simulink model "Model_TranslationEngine64"  (R2022b)
settings: Solver=FixedStepDiscrete  StartTime=0.0  StopTime=5  RelTol=1e-3  EnableMultiTasking=on
InitFcn:
  | % Initialize model
  | ModelSettings=BTConfig.GetModelSettings();
  | 
  | ModelSettings.Validate();
  | 
  | ModelInit;
  | 
  | 
  | % load library data
  | GainLibrary_data;
  | % Load saved values from partition process
  | CapturedConstMask.LoadMapFromFile(bdroot)
StartFcn:
  | % make sure all the simulated RTC requests are found
  | %RTC_SIM_OBJ.ValidateREQs();
undefined symbols (not defined in the file or in its folder): AA, BPLP, Column, NumHFRefBPF, NumHFRefLPF, NumMusicChannels, Row, VolumeMuteConfig
libraries: TuneVar x925, TOP x490, FeaturePath x111, CapturedConstLib x52
(part 5 of 34)

== system Model_TranslationEngine64/ModelPreAmp/DecRate/AudioPilot35/EntertainmentLevelDetection/PreProcessing ==
  FeaturePath : FeaturePath/FeaturePath  FeatureName=LevelDetect  IsGroup=off  GroupNumber=-1  IsModule=off  TriggerInit=[565 224 680 331]
      settings: SourceProductName=Bose Talaria
  MusicDelay : Subsystem
  PreEmphasisShelfFilter : Subsystem  LoadFcn="fprintf(\"\\n ''%s'' block does not support BTC and hence, it will be deprecated soon. Please replace all the active instances of \"\"PooliirwithNonTrivialTranslations\"\" with an equivalent BTC block.\", gcb);"  mask(Bose Pool IIR){maxNumStages=NumInputChannels * Config.ShelfNumStages, numStages=repmat(Config.ShelfNumStages,NumInputChannels,1), sosCoefficients=repmat(Config.ShelfSos,NumInputChannels,1), alias='Default', variantType=Config.LevDetPreEmpPooliirVariant, FeatureName=Preemphasis}
      mask prompts: maxNumStages "Maximum number of stages"; numStages "Number of stages per channel"; sosCoefficients "Coefficient pool"; variantType "Variant"; FeatureName "Filter name/purpose"
      mask init:
      | blkh = gcbh;
      | % Copy discrete mask parameters into a classdef object
      | InnerLinkConfig = PoolIirTunableConfig;
      | InnerLinkConfig.MaxNumStages = maxNumStages;
      | InnerLinkConfig.DefaultNumStages = numStages;
      | InnerLinkConfig.DefaultSosCoefficients = sosCoefficients;
      | InnerLinkConfig.Alias = alias;
      | if(isa(variantType, 'char'))
      |     InnerLinkConfig.SelectVariant(variantType);
      | else
      |     error("Please specify the variant in a character format for ''%s''", gcb);
      | end
      mask TypeOptions FeatureName: InnerLink/FeatureName
      mask Display:
      | [path,w,h] = IconIIR_Mask();
      | 
      | % work in pixels since the icon does not scale
      | pos = get(gcbh,'position');
      | bw = pos(3) - pos(1);
      | bh = pos(4) - pos(2);
      | 
      | % Draw centered icon
      | xAdj = bw/2 - w/2;
      | yAdj = bh/2 - h/2 + 4;
      | for i=1:length(path)
      | %     patch(path(i).x+xAdj, path(i).y+yAdj, path(i).rgb);
      |     plot(path(i).x+xAdj, path(i).y+yAdj);
      | end
      | 
      | % Anchor the corners of the coordinate system
      | patch(0,0,[1 1 1]);
      | patch(bw,bh,[1 1 1]);
      | 
      | % Display some text
      | text(bw/2, 1,'Pool IIR', ...
      |     'horizontalAlignment','center', ...
      |     'VerticalAlignment','bottom');
  SysMax : Subsystem  mask(Talaria Trivial Tune TOP){TriggerInit=[215 414 420 476], TopName=SysMaxDbspl, TuneName=SysMaxDbspl, DataTypeOut=single, MaskValue=Config.MaxDbspl, TunabilityNumber=1, MinValue=[], MaxValue=[], BankNumber=0, PreOverlay=false, PostOverlay=false, UseSameName=on}
      mask prompts: TriggerInit "Hidden: MoveFcn redraw"; TopName "Name:"; TuneName "Name of TuneVar:"; DataTypeOut "Data type:"; MaskValue "Default Value:"; TunabilityNumber "Tunability:"; MinValue "Min Value:"; MaxValue "Max Value:"; BankNumber "Target memory bank number:"; PreOverlay "Requires pre-overlay action:"; PostOverlay "Requires post-overlay action:"; UseSameName "Use same name for tune variable and TOP"
      mask help: The TuneTOP block encapsultes a Target Overlay Parameter, a Tune Variable, and a Trivial Translation between them.
      mask init:
      | [ok,activeTopPath,activeTunePath] = TuneTOP_Mask.Init(gcbh);
      settings: MoveFcn=TuneTOP_Mask.CB_TriggerInit(gcbh);
      mask Callback TriggerInit: TuneTOP_Mask.CB_TriggerInit(gcbh);
      mask TypeOptions TopName: TOP/TopName
      mask TypeOptions TuneName: Tune Variable/TuneName
      mask TypeOptions DataTypeOut: TOP/DataTypeOut
      mask TypeOptions MaskValue: Tune Variable/MaskValue
      mask TypeOptions TunabilityNumber: Tune Variable/TunabilityNumber
      mask Callback TunabilityNumber: TuneVarMask.CB_TunabilityNumber(gcbh);
      mask TypeOptions MinValue: Tune Variable/MinValue
      mask TypeOptions MaxValue: Tune Variable/MaxValue
      mask TypeOptions BankNumber: TOP/BankNumber
      mask TypeOptions PreOverlay: TOP/PreOverlay
      mask TypeOptions PostOverlay: TOP/PostOverlay
      mask Callback UseSameName: TuneTOP_Mask.CB_UseSameName(gcbh);
      mask DialogControl toolPanel Prompt: Tuning Tool Hints
      mask DialogControl DescriptionGroup Prompt: Description
      mask DialogControl EditDescription Prompt: Edit Description
      mask DialogControl EditDescription Callback: TuneTOP_Mask.CB_EditDescription(gcbh);
      mask DialogControl TunabilityText Prompt: Easy: Changes nearly every tuning.
      mask DialogControl AdvancedPanel Prompt: Advanced
      mask DialogControl ConvertToFullTranslation Prompt: Irreversible conversion to full translation
      mask DialogControl ConvertToFullTranslation Callback: TuneTOP_Mask.CB_ConvertToFullTranslation(gcbh);
      mask DialogControl ErrorContainer Prompt: Error Messages
      mask Display:
      | % retrieve icon definition
      | [path,w,h] = TuneTOP_Mask.Icon();
      | 
      | % retrieve the block's pixel size
      | pos = get(gcbh,'position');
      | bw = pos(3) - pos(1);
      | bh = pos(4) - pos(2);
      | 
      | % draw centered icon
      | xAdj = bw/2 - w/2 + 5;
      | yAdj = bh/2 - h/2 + 4;
      | for i=1:length(path)
      | 	patch(path(i).x+xAdj, path(i).y+yAdj, path(i).rgb);
      | end
      | 
      | % show the top name or an X
      | if (exist('ok','var') && ok)
      | 	text(bw*0.5, bh*0.2, activeTopPath, 'horizontalAlignment', 'center');
      | 	patch(0,0,[1 1 1]);
      | 	patch(bw,bh,[1 1 1]);
      | else
      | 	tx=bw*0.03;
      | 	ty=bh*0.03;
      | 	patch([0 tx bw bw-tx], [ty 0 bh-ty bh], [1 0 0]);
      | 	patch([0 bw-tx bw tx], [bh-ty 0 ty bh], [1 0 0]);
      | end

== system Model_TranslationEngine64/ModelPreAmp/DecRate/AudioPilot35/Volume/Index2DbTable ==
  TOP_GainDB : TOP/TOP  TriggerInit=[635 177 785 233]  TopName=Table_dB  DataTypeOut=Inherit: Same as input  BankNumber=Config.BankNumber  PreOverlay=false  PostOverlay=false  Role=Automatic
      settings: SourceProductName=Bose Talaria
  TOP_Index : TOP/TOP  TriggerInit=[635 97 785 153]  TopName=Table_Idx  DataTypeOut=Inherit: Same as input  BankNumber=Config.BankNumber  PreOverlay=false  PostOverlay=false  Role=Automatic
      settings: SourceProductName=Bose Talaria
  TranslateTrigger1 : TuneVar/TranslateTrigger  TriggerInit=[491 -5 529 45]
      settings: SourceProductName=Bose Talaria
  TuneTOP : Subsystem  Description=Variable limits the maximum *dB offset* which will be applied to the gain as part of table lookup. It does *not* directly impact the maximum gain applied, only the maximum dB offset.  mask(Talaria Trivial Tune TOP){TriggerInit=[670 347 840 403], TopName=maxgain, TuneName=maxgain, DataTypeOut=single, MaskValue=Config.DefaultMaxDbOffset, TunabilityNumber=1, MinValue=[], MaxValue=[], BankNumber=0, PreOverlay=false, PostOverlay=false, UseSameName=on}
      mask prompts: TriggerInit "Hidden: MoveFcn redraw"; TopName "Name:"; TuneName "Name of TuneVar:"; DataTypeOut "Data type:"; MaskValue "Default Value:"; TunabilityNumber "Tunability:"; MinValue "Min Value:"; MaxValue "Max Value:"; BankNumber "Target memory bank number:"; PreOverlay "Requires pre-overlay action:"; PostOverlay "Requires post-overlay action:"; UseSameName "Use same name for tune variable and TOP"
      mask help: The TuneTOP block encapsultes a Target Overlay Parameter, a Tune Variable, and a Trivial Translation between them.
      mask init:
      | [ok,activeTopPath,activeTunePath] = TuneTOP_Mask.Init(gcbh);
      settings: MoveFcn=TuneTOP_Mask.CB_TriggerInit(gcbh);
      mask Callback TriggerInit: TuneTOP_Mask.CB_TriggerInit(gcbh);
      mask TypeOptions TopName: TOP/TopName
      mask TypeOptions TuneName: Tune Variable/TuneName
      mask TypeOptions DataTypeOut: TOP/DataTypeOut
      mask TypeOptions MaskValue: Tune Variable/MaskValue
      mask TypeOptions TunabilityNumber: Tune Variable/TunabilityNumber
      mask Callback TunabilityNumber: TuneVarMask.CB_TunabilityNumber(gcbh);
      mask TypeOptions MinValue: Tune Variable/MinValue
      mask TypeOptions MaxValue: Tune Variable/MaxValue
      mask TypeOptions BankNumber: TOP/BankNumber
      mask TypeOptions PreOverlay: TOP/PreOverlay
      mask TypeOptions PostOverlay: TOP/PostOverlay
      mask Callback UseSameName: TuneTOP_Mask.CB_UseSameName(gcbh);
      mask DialogControl toolPanel Prompt: Tuning Tool Hints
      mask DialogControl DescriptionGroup Prompt: Description
      mask DialogControl EditDescription Prompt: Edit Description
      mask DialogControl EditDescription Callback: TuneTOP_Mask.CB_EditDescription(gcbh);
      mask DialogControl TunabilityText Prompt: Easy: Changes nearly every tuning.
      mask DialogControl AdvancedPanel Prompt: Advanced
      mask DialogControl ConvertToFullTranslation Prompt: Irreversible conversion to full translation
      mask DialogControl ConvertToFullTranslation Callback: TuneTOP_Mask.CB_ConvertToFullTranslation(gcbh);
      mask DialogControl ErrorContainer Prompt: Error Messages
      mask Display:
      | % retrieve icon definition
      | [path,w,h] = TuneTOP_Mask.Icon();
      | 
      | % retrieve the block's pixel size
      | pos = get(gcbh,'position');
      | bw = pos(3) - pos(1);
      | bh = pos(4) - pos(2);
      | 
      | % draw centered icon
      | xAdj = bw/2 - w/2 + 5;
      | yAdj = bh/2 - h/2 + 4;
      | for i=1:length(path)
      | 	patch(path(i).x+xAdj, path(i).y+yAdj, path(i).rgb);
      | end
      | 
      | % show the top name or an X
      | if (exist('ok','var') && ok)
      | 	text(bw*0.5, bh*0.2, activeTopPath, 'horizontalAlignment', 'center');
      | 	patch(0,0,[1 1 1]);
      | 	patch(bw,bh,[1 1 1]);
      | else
      | 	tx=bw*0.03;
      | 	ty=bh*0.03;
      | 	patch([0 tx bw bw-tx], [ty 0 bh-ty bh], [1 0 0]);
      | 	patch([0 bw-tx bw tx], [bh-ty 0 ty bh], [1 0 0]);
      | end
  TuneVar_Table : TuneVar/TuneVar  Description=|  TuneName=Table  SpecifyMaxSize=on  VariableDim=1 (Row)  MaxSize=[Config.MaximumTablePoints 2]  TunabilityNumber=2  MinValue=[0;-100]  MaxValue=[1;0]  TriggerInit=[190 140 360 190]  MaskValue=Config.DefaultTable
      | <HTML>Gain table maps index to gain.
      | The index values are <FONT color="red">normalized</Font> floats between 0 and 1 while the gains are in dB (i.e. 0 implies no attenuation).
      | </html>
      settings: SourceProductName=Bose Talaria
  table translation : MATLAB Function  TreatAsAtomicUnit=on
  wires:
  table translation/2(Table_dB) -> TOP_GainDB/1
  table translation/1(Table_Idx) -> TOP_Index/1
  TranslateTrigger1/1 -> table translation/Trigger
  TuneVar_Table/1 -> table translation/1(Table)  "Table"

== system Model_TranslationEngine64/ModelPreAmp/DecRate/AudioPilot35/Volume/TuneVarRampTimeMs ==
  TOP : TOP/TOP  TriggerInit=[440 20 585 80]  TopName=RampTime  DataTypeOut=single  BankNumber=BankNumber  PreOverlay=PreOverlay  PostOverlay=PostOverlay  Role=Automatic
      settings: SourceProductName=Bose Talaria
  TrivialTranslation : TuneVar/TrivialTranslation  TriggerInit=[300 28 350 72]
      settings: SourceProductName=Bose Talaria
  Tune Variable : TuneVar/TuneVar  TuneName=RampTime  SpecifyMaxSize=off  VariableDim=1 (Row)  MaxSize=[1 1]  TunabilityNumber=1  MinValue=MinValue  MaxValue=MaxValue  TriggerInit=[20 25 190 75]  MaskValue=MaskValue
      settings: SourceProductName=Bose Talaria
  wires:
  Tune Variable/1 -> TrivialTranslation/1  "RampTime"
  TrivialTranslation/1 -> TOP/1

== system Model_TranslationEngine64/ModelPreAmp/DecRate/Medusa5H1/Balance/Balance ==
  Captured Tune Const : CapturedConstLib/CapturedConst  TriggerInit=[700 257 800 293]  Role=Automatic
      settings: SourceProductName=Bose Talaria
  FeaturePath : FeaturePath/FeaturePath  FeatureName=Balance_Cfg  IsGroup=off  GroupNumber=-1  IsModule=off  TriggerInit=[-435 -186 -320 -79]
      settings: SourceProductName=Bose Talaria
  TOP : TOP/TOP  TriggerInit=[1095 215 1240 275]  TopName=ChanRampMap  DataTypeOut=single  BankNumber=0  PreOverlay=false  PostOverlay=false  Role=Automatic
      settings: SourceProductName=Bose Talaria
  TranslateTrigger : TuneVar/TranslateTrigger  TriggerInit=[951 105 989 160]
      settings: SourceProductName=Bose Talaria
  TuneVarBoostDisable : Subsystem  Description=Specifies the 'boost' value to be applied to the channels towards which the balance is moved. A value of '1' indicates no 'boost' (0 dB) ,whereas '0' indicates that the 'boost' must be computed from the 'cut' value (which gets computed from the Balance table). In order to preserve the overall energy, the following formula is used: Boost^2 + Cut^2 = 2.  mask(Talaria Trivial Tune TOP){TriggerInit=[-50 240 120 280], TopName=BoostDisable, TuneName=BoostDisable, DataTypeOut=single, MaskValue=Config.DefaultMaskBoostDisable, TunabilityNumber=2, MinValue=[], MaxValue=[], BankNumber=Config.BankNumber, PreOverlay=false, PostOverlay=false, UseSameName=on}
      mask prompts: TriggerInit "Hidden: MoveFcn redraw"; TopName "Name:"; TuneName "Name of TuneVar:"; DataTypeOut "Data type:"; MaskValue "Default Value:"; TunabilityNumber "Tunability:"; MinValue "Min Value:"; MaxValue "Max Value:"; BankNumber "Target memory bank number:"; PreOverlay "Requires pre-overlay action:"; PostOverlay "Requires post-overlay action:"; UseSameName "Use same name for tune variable and TOP"
      mask help: The TuneTOP block encapsultes a Target Overlay Parameter, a Tune Variable, and a Trivial Translation between them.
      mask init:
      | [ok,activeTopPath,activeTunePath] = TuneTOP_Mask.Init(gcbh);
      settings: MoveFcn=TuneTOP_Mask.CB_TriggerInit(gcbh);
      mask Callback TriggerInit: TuneTOP_Mask.CB_TriggerInit(gcbh);
      mask TypeOptions TopName: TOP/TopName
      mask TypeOptions TuneName: Tune Variable/TuneName
      mask TypeOptions DataTypeOut: TOP/DataTypeOut
      mask TypeOptions MaskValue: Tune Variable/MaskValue
      mask TypeOptions TunabilityNumber: Tune Variable/TunabilityNumber
      mask Callback TunabilityNumber: TuneVarMask.CB_TunabilityNumber(gcbh);
      mask TypeOptions MinValue: Tune Variable/MinValue
      mask TypeOptions MaxValue: Tune Variable/MaxValue
      mask TypeOptions BankNumber: TOP/BankNumber
      mask TypeOptions PreOverlay: TOP/PreOverlay
      mask TypeOptions PostOverlay: TOP/PostOverlay
      mask Callback UseSameName: TuneTOP_Mask.CB_UseSameName(gcbh);
      mask DialogControl toolPanel Prompt: Tuning Tool Hints
      mask DialogControl DescriptionGroup Prompt: Description
      mask DialogControl EditDescription Prompt: Edit Description
      mask DialogControl EditDescription Callback: TuneTOP_Mask.CB_EditDescription(gcbh);
      mask DialogControl TunabilityText Prompt: Easy: Changes nearly every tuning.
      mask DialogControl AdvancedPanel Prompt: Advanced
      mask DialogControl ConvertToFullTranslation Prompt: Irreversible conversion to full translation
      mask DialogControl ConvertToFullTranslation Callback: TuneTOP_Mask.CB_ConvertToFullTranslation(gcbh);
      mask DialogControl ErrorContainer Prompt: Error Messages
      mask Display:
      | % retrieve icon definition
      | [path,w,h] = TuneTOP_Mask.Icon();
      | 
      | % retrieve the block's pixel size
      | pos = get(gcbh,'position');
      | bw = pos(3) - pos(1);
      | bh = pos(4) - pos(2);
      | 
      | % draw centered icon
      | xAdj = bw/2 - w/2 + 5;
      | yAdj = bh/2 - h/2 + 4;
      | for i=1:length(path)
      | 	patch(path(i).x+xAdj, path(i).y+yAdj, path(i).rgb);
      | end
      | 
      | % show the top name or an X
      | if (exist('ok','var') && ok)
      | 	text(bw*0.5, bh*0.2, activeTopPath, 'horizontalAlignment', 'center');
      | 	patch(0,0,[1 1 1]);
      | 	patch(bw,bh,[1 1 1]);
      | else
      | 	tx=bw*0.03;
      | 	ty=bh*0.03;
      | 	patch([0 tx bw bw-tx], [ty 0 bh-ty bh], [1 0 0]);
      | 	patch([0 bw-tx bw tx], [bh-ty 0 ty bh], [1 0 0]);
      | end
  TuneVarChanRampMap : TuneVar/TuneVar  Description=|  TuneName=ChanRampMap  SpecifyMaxSize=off  VariableDim=1 (Row)  MaxSize=[1 1]  TunabilityNumber=2  MinValue=[]  MaxValue=[]  TriggerInit=[630 190 800 240]  MaskValue=Config.DefaultMaskChanRampMap
      | Specifies the ramper to which each channel is mapped. Replace the channel number with:
      | '1' - 'Right'; '2' - 'Left'; '3' - 'Center'. Currently, the 'Center' group is assigned a linear gain of 1.
      settings: SourceProductName=Bose Talaria
  TuneVarOffset : Subsystem  Description=Defines the index at which the Balance is at the center i.e., neither towards the left or right sides.  mask(Talaria Trivial Tune TOP){TriggerInit=[-50 130 120 170], TopName=Offset, TuneName=Offset, DataTypeOut=single, MaskValue=Config.DefaultMaskOffset, TunabilityNumber=3, MinValue=[], MaxValue=[], BankNumber=Config.BankNumber, PreOverlay=false, PostOverlay=false, UseSameName=on}
      mask prompts: TriggerInit "Hidden: MoveFcn redraw"; TopName "Name:"; TuneName "Name of TuneVar:"; DataTypeOut "Data type:"; MaskValue "Default Value:"; TunabilityNumber "Tunability:"; MinValue "Min Value:"; MaxValue "Max Value:"; BankNumber "Target memory bank number:"; PreOverlay "Requires pre-overlay action:"; PostOverlay "Requires post-overlay action:"; UseSameName "Use same name for tune variable and TOP"
      mask help: The TuneTOP block encapsultes a Target Overlay Parameter, a Tune Variable, and a Trivial Translation between them.
      mask init:
      | [ok,activeTopPath,activeTunePath] = TuneTOP_Mask.Init(gcbh);
      settings: MoveFcn=TuneTOP_Mask.CB_TriggerInit(gcbh);
      mask Callback TriggerInit: TuneTOP_Mask.CB_TriggerInit(gcbh);
      mask TypeOptions TopName: TOP/TopName
      mask TypeOptions TuneName: Tune Variable/TuneName
      mask TypeOptions DataTypeOut: TOP/DataTypeOut
      mask TypeOptions MaskValue: Tune Variable/MaskValue
      mask TypeOptions TunabilityNumber: Tune Variable/TunabilityNumber
      mask Callback TunabilityNumber: TuneVarMask.CB_TunabilityNumber(gcbh);
      mask TypeOptions MinValue: Tune Variable/MinValue
      mask TypeOptions MaxValue: Tune Variable/MaxValue
      mask TypeOptions BankNumber: TOP/BankNumber
      mask TypeOptions PreOverlay: TOP/PreOverlay
      mask TypeOptions PostOverlay: TOP/PostOverlay
      mask Callback UseSameName: TuneTOP_Mask.CB_UseSameName(gcbh);
      mask DialogControl toolPanel Prompt: Tuning Tool Hints
      mask DialogControl DescriptionGroup Prompt: Description
      mask DialogControl EditDescription Prompt: Edit Description
      mask DialogControl EditDescription Callback: TuneTOP_Mask.CB_EditDescription(gcbh);
      mask DialogControl TunabilityText Prompt: Easy: Changes nearly every tuning.
      mask DialogControl AdvancedPanel Prompt: Advanced
      mask DialogControl ConvertToFullTranslation Prompt: Irreversible conversion to full translation
      mask DialogControl ConvertToFullTranslation Callback: TuneTOP_Mask.CB_ConvertToFullTranslation(gcbh);
      mask DialogControl ErrorContainer Prompt: Error Messages
      mask Display:
      | % retrieve icon definition
      | [path,w,h] = TuneTOP_Mask.Icon();
      | 
      | % retrieve the block's pixel size
      | pos = get(gcbh,'position');
      | bw = pos(3) - pos(1);
      | bh = pos(4) - pos(2);
      | 
      | % draw centered icon
      | xAdj = bw/2 - w/2 + 5;
      | yAdj = bh/2 - h/2 + 4;
      | for i=1:length(path)
      | 	patch(path(i).x+xAdj, path(i).y+yAdj, path(i).rgb);
      | end
      | 
      | % show the top name or an X
      | if (exist('ok','var') && ok)
      | 	text(bw*0.5, bh*0.2, activeTopPath, 'horizontalAlignment', 'center');
      | 	patch(0,0,[1 1 1]);
      | 	patch(bw,bh,[1 1 1]);
      | else
      | 	tx=bw*0.03;
      | 	ty=bh*0.03;
      | 	patch([0 tx bw bw-tx], [ty 0 bh-ty bh], [1 0 0]);
      | 	patch([0 bw-tx bw tx], [bh-ty 0 ty bh], [1 0 0]);
      | end
  TuneVarRampTime : Subsystem  Description=Specifies the default ramp time for the rampers.  mask(Talaria Trivial Tune TOP){TriggerInit=[630 -80 800 -40], TopName=RampTime, TuneName=RampTime, DataTypeOut=single, MaskValue=30, TunabilityNumber=2, MinValue=[], MaxValue=[], BankNumber=Config.BankNumber, PreOverlay=false, PostOverlay=false, UseSameName=on}
      mask prompts: TriggerInit "Hidden: MoveFcn redraw"; TopName "Name:"; TuneName "Name of TuneVar:"; DataTypeOut "Data type:"; MaskValue "Default Value:"; TunabilityNumber "Tunability:"; MinValue "Min Value:"; MaxValue "Max Value:"; BankNumber "Target memory bank number:"; PreOverlay "Requires pre-overlay action:"; PostOverlay "Requires post-overlay action:"; UseSameName "Use same name for tune variable and TOP"
      mask help: The TuneTOP block encapsultes a Target Overlay Parameter, a Tune Variable, and a Trivial Translation between them.
      mask init:
      | [ok,activeTopPath,activeTunePath] = TuneTOP_Mask.Init(gcbh);
      settings: MoveFcn=TuneTOP_Mask.CB_TriggerInit(gcbh);
      mask Callback TriggerInit: TuneTOP_Mask.CB_TriggerInit(gcbh);
      mask TypeOptions TopName: TOP/TopName
      mask TypeOptions TuneName: Tune Variable/TuneName
      mask TypeOptions DataTypeOut: TOP/DataTypeOut
      mask TypeOptions MaskValue: Tune Variable/MaskValue
      mask TypeOptions TunabilityNumber: Tune Variable/TunabilityNumber
      mask Callback TunabilityNumber: TuneVarMask.CB_TunabilityNumber(gcbh);
      mask TypeOptions MinValue: Tune Variable/MinValue
      mask TypeOptions MaxValue: Tune Variable/MaxValue
      mask TypeOptions BankNumber: TOP/BankNumber
      mask TypeOptions PreOverlay: TOP/PreOverlay
      mask TypeOptions PostOverlay: TOP/PostOverlay
      mask Callback UseSameName: TuneTOP_Mask.CB_UseSameName(gcbh);
      mask DialogControl toolPanel Prompt: Tuning Tool Hints
      mask DialogControl DescriptionGroup Prompt: Description
      mask DialogControl EditDescription Prompt: Edit Description
      mask DialogControl EditDescription Callback: TuneTOP_Mask.CB_EditDescription(gcbh);
      mask DialogControl TunabilityText Prompt: Easy: Changes nearly every tuning.
      mask DialogControl AdvancedPanel Prompt: Advanced
      mask DialogControl ConvertToFullTranslation Prompt: Irreversible conversion to full translation
      mask DialogControl ConvertToFullTranslation Callback: TuneTOP_Mask.CB_ConvertToFullTranslation(gcbh);
      mask DialogControl ErrorContainer Prompt: Error Messages
      mask Display:
      | % retrieve icon definition
      | [path,w,h] = TuneTOP_Mask.Icon();
      | 
      | % retrieve the block's pixel size
      | pos = get(gcbh,'position');
      | bw = pos(3) - pos(1);
      | bh = pos(4) - pos(2);
      | 
      | % draw centered icon
      | xAdj = bw/2 - w/2 + 5;
      | yAdj = bh/2 - h/2 + 4;
      | for i=1:length(path)
      | 	patch(path(i).x+xAdj, path(i).y+yAdj, path(i).rgb);
      | end
      | 
      | % show the top name or an X
      | if (exist('ok','var') && ok)
      | 	text(bw*0.5, bh*0.2, activeTopPath, 'horizontalAlignment', 'center');
      | 	patch(0,0,[1 1 1]);
      | 	patch(bw,bh,[1 1 1]);
      | else
      | 	tx=bw*0.03;
      | 	ty=bh*0.03;
      | 	patch([0 tx bw bw-tx], [ty 0 bh-ty bh], [1 0 0]);
      | 	patch([0 bw-tx bw tx], [bh-ty 0 ty bh], [1 0 0]);
      | end
  TuneVarSilentBass : Subsystem  mask(Talaria Trivial Tune TOP){TriggerInit=[-50 452 120 508], TopName=SleepingBeautyMutesBass, TuneName=SleepingBeautyMutesBass, DataTypeOut=single, MaskValue=Config.DefaultMaskSilentExtremeBass, TunabilityNumber=1, MinValue=[], MaxValue=[], BankNumber=Config.BankNumber, PreOverlay=false, PostOverlay=false, UseSameName=on}
      mask prompts: TriggerInit "Hidden: MoveFcn redraw"; TopName "Name:"; TuneName "Name of TuneVar:"; DataTypeOut "Data type:"; MaskValue "Default Value:"; TunabilityNumber "Tunability:"; MinValue "Min Value:"; MaxValue "Max Value:"; BankNumber "Target memory bank number:"; PreOverlay "Requires pre-overlay action:"; PostOverlay "Requires post-overlay action:"; UseSameName "Use same name for tune variable and TOP"
      mask help: The TuneTOP block encapsultes a Target Overlay Parameter, a Tune Variable, and a Trivial Translation between them.
      mask init:
      | [ok,activeTopPath,activeTunePath] = TuneTOP_Mask.Init(gcbh);
      settings: MoveFcn=TuneTOP_Mask.CB_TriggerInit(gcbh);
      mask Callback TriggerInit: TuneTOP_Mask.CB_TriggerInit(gcbh);
      mask TypeOptions TopName: TOP/TopName
      mask TypeOptions TuneName: Tune Variable/TuneName
      mask TypeOptions DataTypeOut: TOP/DataTypeOut
      mask TypeOptions MaskValue: Tune Variable/MaskValue
      mask TypeOptions TunabilityNumber: Tune Variable/TunabilityNumber
      mask Callback TunabilityNumber: TuneVarMask.CB_TunabilityNumber(gcbh);
      mask TypeOptions MinValue: Tune Variable/MinValue
      mask TypeOptions MaxValue: Tune Variable/MaxValue
      mask TypeOptions BankNumber: TOP/BankNumber
      mask TypeOptions PreOverlay: TOP/PreOverlay
      mask TypeOptions PostOverlay: TOP/PostOverlay
      mask Callback UseSameName: TuneTOP_Mask.CB_UseSameName(gcbh);
      mask DialogControl toolPanel Prompt: Tuning Tool Hints
      mask DialogControl DescriptionGroup Prompt: Description
      mask DialogControl EditDescription Prompt: Edit Description
      mask DialogControl EditDescription Callback: TuneTOP_Mask.CB_EditDescription(gcbh);
      mask DialogControl TunabilityText Prompt: Easy: Changes nearly every tuning.
      mask DialogControl AdvancedPanel Prompt: Advanced
      mask DialogControl ConvertToFullTranslation Prompt: Irreversible conversion to full translation
      mask DialogControl ConvertToFullTranslation Callback: TuneTOP_Mask.CB_ConvertToFullTranslation(gcbh);
      mask DialogControl ErrorContainer Prompt: Error Messages
      mask Display:
      | % retrieve icon definition
      | [path,w,h] = TuneTOP_Mask.Icon();
      | 
      | % retrieve the block's pixel size
      | pos = get(gcbh,'position');
      | bw = pos(3) - pos(1);
      | bh = pos(4) - pos(2);
      | 
      | % draw centered icon
      | xAdj = bw/2 - w/2 + 5;
      | yAdj = bh/2 - h/2 + 4;
      | for i=1:length(path)
      | 	patch(path(i).x+xAdj, path(i).y+yAdj, path(i).rgb);
      | end
      | 
      | % show the top name or an X
      | if (exist('ok','var') && ok)
      | 	text(bw*0.5, bh*0.2, activeTopPath, 'horizontalAlignment', 'center');
      | 	patch(0,0,[1 1 1]);
      | 	patch(bw,bh,[1 1 1]);
      | else
      | 	tx=bw*0.03;
      | 	ty=bh*0.03;
      | 	patch([0 tx bw bw-tx], [ty 0 bh-ty bh], [1 0 0]);
      | 	patch([0 bw-tx bw tx], [bh-ty 0 ty bh], [1 0 0]);
      | end
  TuneVarSilentExtreme : Subsystem  Description=|  mask(Talaria Trivial Tune TOP){TriggerInit=[-50 350 120 390], TopName=EnableSilentExtreme, TuneName=EnableSilentExtreme, DataTypeOut=single, MaskValue=Config.DefaultMaskSilentExtreme, TunabilityNumber=2, MinValue=[], MaxValue=[], BankNumber=Config.BankNumber, PreOverlay=false, PostOverlay=false, UseSameName=on}
      | 0 implies no special handling
      | 1 implies special muting of the "cut" channel, in addition to the center channels) when the input control is at its extremes (lowest or highest index is provided)
      mask prompts: TriggerInit "Hidden: MoveFcn redraw"; TopName "Name:"; TuneName "Name of TuneVar:"; DataTypeOut "Data type:"; MaskValue "Default Value:"; TunabilityNumber "Tunability:"; MinValue "Min Value:"; MaxValue "Max Value:"; BankNumber "Target memory bank number:"; PreOverlay "Requires pre-overlay action:"; PostOverlay "Requires post-overlay action:"; UseSameName "Use same name for tune variable and TOP"
      mask help: The TuneTOP block encapsultes a Target Overlay Parameter, a Tune Variable, and a Trivial Translation between them.
      mask init:
      | [ok,activeTopPath,activeTunePath] = TuneTOP_Mask.Init(gcbh);
      settings: MoveFcn=TuneTOP_Mask.CB_TriggerInit(gcbh);
      mask Callback TriggerInit: TuneTOP_Mask.CB_TriggerInit(gcbh);
      mask TypeOptions TopName: TOP/TopName
      mask TypeOptions TuneName: Tune Variable/TuneName
      mask TypeOptions DataTypeOut: TOP/DataTypeOut
      mask TypeOptions MaskValue: Tune Variable/MaskValue
      mask TypeOptions TunabilityNumber: Tune Variable/TunabilityNumber
      mask Callback TunabilityNumber: TuneVarMask.CB_TunabilityNumber(gcbh);
      mask TypeOptions MinValue: Tune Variable/MinValue
      mask TypeOptions MaxValue: Tune Variable/MaxValue
      mask TypeOptions BankNumber: TOP/BankNumber
      mask TypeOptions PreOverlay: TOP/PreOverlay
      mask TypeOptions PostOverlay: TOP/PostOverlay
      mask Callback UseSameName: TuneTOP_Mask.CB_UseSameName(gcbh);
      mask DialogControl toolPanel Prompt: Tuning Tool Hints
      mask DialogControl DescriptionGroup Prompt: Description
      mask DialogControl EditDescription Prompt: Edit Description
      mask DialogControl EditDescription Callback: TuneTOP_Mask.CB_EditDescription(gcbh);
      mask DialogControl TunabilityText Prompt: Easy: Changes nearly every tuning.
      mask DialogControl AdvancedPanel Prompt: Advanced
      mask DialogControl ConvertToFullTranslation Prompt: Irreversible conversion to full translation
      mask DialogControl ConvertToFullTranslation Callback: TuneTOP_Mask.CB_ConvertToFullTranslation(gcbh);
      mask DialogControl ErrorContainer Prompt: Error Messages
      mask Display:
      | % retrieve icon definition
      | [path,w,h] = TuneTOP_Mask.Icon();
      | 
      | % retrieve the block's pixel size
      | pos = get(gcbh,'position');
      | bw = pos(3) - pos(1);
      | bh = pos(4) - pos(2);
      | 
      | % draw centered icon
      | xAdj = bw/2 - w/2 + 5;
      | yAdj = bh/2 - h/2 + 4;
      | for i=1:length(path)
      | 	patch(path(i).x+xAdj, path(i).y+yAdj, path(i).rgb);
      | end
      | 
      | % show the top name or an X
      | if (exist('ok','var') && ok)
      | 	text(bw*0.5, bh*0.2, activeTopPath, 'horizontalAlignment', 'center');
      | 	patch(0,0,[1 1 1]);
      | 	patch(bw,bh,[1 1 1]);
      | else
      | 	tx=bw*0.03;
      | 	ty=bh*0.03;
      | 	patch([0 tx bw bw-tx], [ty 0 bh-ty bh], [1 0 0]);
      | 	patch([0 bw-tx bw tx], [bh-ty 0 ty bh], [1 0 0]);
      | end
  TuneVarTable : Subsystem  Description=Given in dB, sets the maximum impact of balance processing among channels.
  channel_ramper_translation : MATLAB Function  TreatAsAtomicUnit=on
  wires:
  TranslateTrigger/1 -> channel_ramper_translation/Trigger
  channel_ramper_translation/1(ChanRampMap) -> TOP/1
  TuneVarChanRampMap/1 -> channel_ramper_translation/1(TuneChanRampMap)  "ChanRampMap"
  Captured Tune Const/1 -> channel_ramper_translation/2(channelCount)

== system Model_TranslationEngine64/ModelPreAmp/DecRate/Medusa5H1/MedusaHoligram/Medusa5H1 Part 1 ==
  Bass Manager Stereo : Subsystem  RTWFileName=MedusaBassManager  mask(Bass Manager){Config=ConfigBTC.BassManager}
      mask prompts: Config "MedusaBassManagerConfig"
      mask help:
      | The block primarily performs the following functions:
      | 1. Band Separation: Separates the bass content from the higher frequency content
      | 2. Provide bass enhancement and distribute the bass content throughout the channels.
      |
      | Input:
      | The block can support stereo, 5.1 and 5.1.4 input formats. It accepts the inputs in the following order:
      | 1. Stereo: L, R
      | 2. 5.1: L, R, Ls, Rs, C, LFE
      | 3. 5.1.4: L, R, Ls, Rs, C, LFE, LTF, RTF, LTB, RTB
      |
      | Output:
      | The block offers two multi-channel outputs.
      | 1. Bass content: Lbass, Rbass
      | 2. Highpass content: High frequency content in the following order
      |     (a) Stereo configuration: L, R
      |     (b) 5.1 configuration: C*, L, R, Ls, Rs
      |     (c) 5.1.4 configuration: C*, L, R, Ls, Rs, LTF, RTF, LTB, RTB
      |
      | For more information and sample generation of config object, please see 'Help'.
      mask init:
      | blkh=gcbh;
      | Config=BTConfig.Assert(blkh,Config);
      | 
      | Config.Validate();
      | Config.DoMaskInit(blkh);
      settings: RTWSystemCode=Nonreusable function  RTWFileNameOpts=User specified  FunctionWithSeparateData=on
      mask Help:
      | <b>Background</b>
      | 
      | The LPF and HPF are 5th-order Butterworth filters. These act as band separation filters (crossover filter or XOF). The default cross-over frequency is 90 Hz.
      | 
      | For discrete inputs, the LFE content is mixed to C before performing high-pass filtering in order to preserve the LFE content from 90Hz-120Hz.
      | 
      | 
      | <b>Usage</b>
      | 
      | BassManager =  MedusaBassManagerConfig;
  CAE Treble Boost : Subsystem  Variant=on
  TuneVar : TuneVar/TuneVar  Description=|  TuneName=SurroundOn  SpecifyMaxSize=off  VariableDim=1 (Row)  MaxSize=[1 1]  TunabilityNumber=1  MinValue=[]  MaxValue=[]  TriggerInit=[235 97 315 133]  MaskValue=ConfigBTC.TuneVarBmSurroundOn
      | General surround control parameter
      | STEREO_MODE = 0
      | SURROUND_PASSTHRU_MODE = 1
      | MEDUSA_2_CHANNEL_MODE = 2
      | MEDUSA_5_1_MODE = 3
      settings: SourceProductName=Bose Talaria
  wires:
  TuneVar/1 -> Bass Manager Stereo/1(SurroundOn (TuneVar))  "SurroundOn"

== system Model_TranslationEngine64/ModelPreAmp/DecRate/Medusa5H1/MedusaHoligram/Medusa5H1 Part 2 ==
  Alignment Delay : Subsystem  TreatAsAtomicUnit=on
      settings: RTWSystemCode=Nonreusable function  FunctionWithSeparateData=on
  Decimated-Rate FDP : Subsystem  mask(MedusaFdp){Config=ConfigBTC.DeciRateFdp}
      mask prompts: Config "MedusaFdpConfig"
      mask help:
      | See "help" for more information, or run
      | >> help MedusaFdpConfig
      mask init:
      | blkh=gcbh;
      | Config=BTConfig.Assert(blkh,Config);
      | 
      | Config.Validate();
      | Config.DoMaskInit(blkh);
      mask Help: eval("help MedusaFdpConfig")
  Full-Rate FDP : Subsystem  mask(MedusaFdp){Config=ConfigBTC.FullRateFdp}
      mask prompts: Config "MedusaFdpConfig"
      mask help:
      | See "help" for more information, or run
      | >> help MedusaFdpConfig
      mask init:
      | blkh=gcbh;
      | Config=BTConfig.Assert(blkh,Config);
      | 
      | Config.Validate();
      | Config.DoMaskInit(blkh);
      mask Help: eval("help MedusaFdpConfig")
  Mono Detector : Subsystem  mask(Mono Detector){Config=ConfigBTC.MonoDetector}
      mask prompts: Config "MedusaMonoDetectorConfig"
      mask help:
      | This block detects if given stereo input (L, R) is stereo. The output isStereo is used to enable/disable Spatial Unmasker in Medusa system. When the block is put to passthrough by tuning, the default output is set to 'true'.
      |
      | Configuration struct needs to define the below fields with the exact names which are used inside the block.
      |
      | decimationFactor: decimation factor
      | maxZeroLevelCount: maximum number of zero signals in a row before reset
      | hpfOrder: order of highpass filter
      | maxNumStages: maximum of sos for both L and R highpass filter
      | numChannels: number of channels
      |
      | For more information and sample generation of config struct, please see 'Help'.
      mask init:
      | blkh=gcbh;
      | Config=BTConfig.Assert(blkh,Config);
      | 
      | Config.Validate();
      mask Help:
      | Model that uses Mono Detector block need to call MonoDetectorInit(config) to generate <i>MonoDetectorConfigStruct</i> and <i>MonoDetectorTunable</i> bus object in base workspace.
      | 
      | <b>Sample usage:</b>
      | 
      | MedusaConfig = generateMedusaConfig(auto_gen_sys_defs);
      | MonoDetectorInit(MedusaConfig);
      | or
      | DefaultMedusaConfig = generateMedusaConfig();
      | MonoDetectorInit(DefaultMedusaConfig);
  SPUM Decay Estimate : Subsystem  mask{configStruct=config.FRFDPConfig}
      mask prompts: configStruct "Config struct name:"
      mask init:
      | decayConst = configStruct.decayEstimateConst;
      | frameSize = configStruct.frameSize * 4;

== system Model_TranslationEngine64/ModelPreAmp/DecRate/Medusa5H1/MedusaHoligram/Medusa5H1 Part 3 ==
  On : Subsystem

== system Model_TranslationEngine64/ModelPreAmp/DecRate/Medusa5H1/MedusaHoligram/Medusa5H1 Part 4 ==
  On : Subsystem

== system Model_TranslationEngine64/ModelPreAmp/DecRate/Medusa5H1/MedusaHoligram/Medusa5H1 Part 6 ==
  Speaker Delay Tune : Subsystem

== system Model_TranslationEngine64/ModelPreAmp/DecRate/Medusa5H1/MedusaPostHoligram/MedusaPostHoligram ==
  FeaturePath : FeaturePath/FeaturePath  FeatureName=Medusa  IsGroup=off  GroupNumber=-1  IsModule=off  TriggerInit=[810 309 925 416]
      settings: SourceProductName=Bose Talaria
  On : Subsystem

== system Model_TranslationEngine64/ModelPreAmp/DecRate/Medusa5H1/NearWiggleFilters/NEAR ==
  NearOff : Subsystem  VariantControl=0 == Config.NearEnable
  NearOn : Subsystem  VariantControl=0 ~= Config.NearEnable

== system Model_TranslationEngine64/ModelPreAmp/DecRate/Medusa5H1/SleepingBeauty/SleepingBeauty ==
  Bypass : Subsystem  TreatAsAtomicUnit=on  VariantControl=Config.SleepingBeautyEnabled == 0
      settings: RTWSystemCode=Nonreusable function  RTWFcnNameOpts=Use subsystem name  RTWFileNameOpts=Use subsystem name
  Enabled : Subsystem  TreatAsAtomicUnit=on  VariantControl=(default)
      settings: RTWSystemCode=Nonreusable function  RTWFcnNameOpts=Use subsystem name  RTWFileNameOpts=Use subsystem name

== system Model_TranslationEngine64/ModelPreAmp/DecRate/Medusa5H1/VLS/Crosstalk Cancellation ==
  FeaturePath : FeaturePath/FeaturePath  FeatureName=XtalkCancellation  IsGroup=off  GroupNumber=-1  IsModule=off  TriggerInit=[365 -126 480 -19]
      settings: SourceProductName=Bose Talaria
  Pooliir with Non-Trivial Translations : Subsystem  LoadFcn="fprintf(\"\\n ''%s'' block does not support BTC and hence, it will be deprecated soon. Please replace all the active instances of \"\"PooliirwithNonTrivialTranslations\"\" with an equivalent BTC block.\", gcb);"  mask(Bose Pool IIR){maxNumStages=IIR.maxNumStages, numStages=IIR.numStages, sosCoefficients=IIR.coeffs, alias=IIR.alias, variantType=IIR.variantSelect, FeatureName=IIR}
      mask prompts: maxNumStages "Maximum number of stages"; numStages "Number of stages per channel"; sosCoefficients "Coefficient pool"; variantType "Variant"; FeatureName "Filter name/purpose"
      mask init: same as Model_TranslationEngine64/ModelPreAmp/DecRate/AudioPilot35/EntertainmentLevelDetection/PreProcessing/PreEmphasisShelfFilter
      mask TypeOptions FeatureName: InnerLink/FeatureName
      mask Display:
      | [path,w,h] = IconIIR_Mask();
      | 
      | % work in pixels since the icon does not scale
      | pos = get(gcbh,'position');
      | bw = pos(3) - pos(1);
      | bh = pos(4) - pos(2);
      | 
      | % Draw centered icon
      | xAdj = bw/2 - w/2;
      | yAdj = bh/2 - h/2 + 4;
      | for i=1:length(path)
      | %     patch(path(i).x+xAdj, path(i).y+yAdj, path(i).rgb);
      |     plot(path(i).x+xAdj, path(i).y+yAdj);
      | end
      | 
      | % Anchor the corners of the coordinate system
      | patch(0,0,[1 1 1]);
      | patch(bw,bh,[1 1 1]);
      | 
      | % Display some text
      | text(bw/2, 1,'Pool IIR', ...
      |     'horizontalAlignment','center', ...
      |     'VerticalAlignment','bottom');
  TuneTOP : Subsystem  mask(Talaria Trivial Tune TOP){TriggerInit=[535 102 705 158], TopName=Delay, TuneName=Delay, DataTypeOut=int32, MaskValue=configStruct.delayDefault, TunabilityNumber=1, MinValue=[], MaxValue=[], BankNumber=0, PreOverlay=false, PostOverlay=false, UseSameName=on}
      mask prompts: TriggerInit "Hidden: MoveFcn redraw"; TopName "Name:"; TuneName "Name of TuneVar:"; DataTypeOut "Data type:"; MaskValue "Default Value:"; TunabilityNumber "Tunability:"; MinValue "Min Value:"; MaxValue "Max Value:"; BankNumber "Target memory bank number:"; PreOverlay "Requires pre-overlay action:"; PostOverlay "Requires post-overlay action:"; UseSameName "Use same name for tune variable and TOP"
      mask help: The TuneTOP block encapsultes a Target Overlay Parameter, a Tune Variable, and a Trivial Translation between them.
      mask init:
      | [ok,activeTopPath,activeTunePath] = TuneTOP_Mask.Init(gcbh);
      settings: MoveFcn=TuneTOP_Mask.CB_TriggerInit(gcbh);
      mask Callback TriggerInit: TuneTOP_Mask.CB_TriggerInit(gcbh);
      mask TypeOptions TopName: TOP/TopName
      mask TypeOptions TuneName: Tune Variable/TuneName
      mask TypeOptions DataTypeOut: TOP/DataTypeOut
      mask TypeOptions MaskValue: Tune Variable/MaskValue
      mask TypeOptions TunabilityNumber: Tune Variable/TunabilityNumber
      mask Callback TunabilityNumber: TuneVarMask.CB_TunabilityNumber(gcbh);
      mask TypeOptions MinValue: Tune Variable/MinValue
      mask TypeOptions MaxValue: Tune Variable/MaxValue
      mask TypeOptions BankNumber: TOP/BankNumber
      mask TypeOptions PreOverlay: TOP/PreOverlay
      mask TypeOptions PostOverlay: TOP/PostOverlay
      mask Callback UseSameName: TuneTOP_Mask.CB_UseSameName(gcbh);
      mask DialogControl toolPanel Prompt: Tuning Tool Hints
      mask DialogControl DescriptionGroup Prompt: Description
      mask DialogControl EditDescription Prompt: Edit Description
      mask DialogControl EditDescription Callback: TuneTOP_Mask.CB_EditDescription(gcbh);
      mask DialogControl TunabilityText Prompt: Easy: Changes nearly every tuning.
      mask DialogControl AdvancedPanel Prompt: Advanced
      mask DialogControl ConvertToFullTranslation Prompt: Irreversible conversion to full translation
      mask DialogControl ConvertToFullTranslation Callback: TuneTOP_Mask.CB_ConvertToFullTranslation(gcbh);
      mask DialogControl ErrorContainer Prompt: Error Messages
      mask DialogControl ErrorText Prompt: Default value cannot be empty. Tune variables must have non-zero dimensions.
      mask Display:
      | % retrieve icon definition
      | [path,w,h] = TuneTOP_Mask.Icon();
      | 
      | % retrieve the block's pixel size
      | pos = get(gcbh,'position');
      | bw = pos(3) - pos(1);
      | bh = pos(4) - pos(2);
      | 
      | % draw centered icon
      | xAdj = bw/2 - w/2 + 5;
      | yAdj = bh/2 - h/2 + 4;
      | for i=1:length(path)
      | 	patch(path(i).x+xAdj, path(i).y+yAdj, path(i).rgb);
      | end
      | 
      | % show the top name or an X
      | if (exist('ok','var') && ok)
      | 	text(bw*0.5, bh*0.2, activeTopPath, 'horizontalAlignment', 'center');
      | 	patch(0,0,[1 1 1]);
      | 	patch(bw,bh,[1 1 1]);
      | else
      | 	tx=bw*0.03;
      | 	ty=bh*0.03;
      | 	patch([0 tx bw bw-tx], [ty 0 bh-ty bh], [1 0 0]);
      | 	patch([0 bw-tx bw tx], [bh-ty 0 ty bh], [1 0 0]);
      | end

== system Model_TranslationEngine64/ModelPreAmp/DecRate/Medusa5H1/VLS/VLS Generation - D ==
  FeaturePath : FeaturePath/FeaturePath  FeatureName=GenerationDrv  IsGroup=off  GroupNumber=-1  IsModule=off  TriggerInit=[120 244 235 351]
      settings: SourceProductName=Bose Talaria
  TOP : TOP/TOP  TriggerInit=[815 370 985 430]  TopName=FIRCoeffs  DataTypeOut=single  BankNumber=1  PreOverlay=false  PostOverlay=false  Role=Automatic
      settings: SourceProductName=Bose Talaria
  TOP2 : TOP/TOP  TriggerInit=[815 465 985 525]  TopName=PaddedFilterLengths  DataTypeOut=uint32  BankNumber=0  PreOverlay=false  PostOverlay=false  Role=Automatic
      settings: SourceProductName=Bose Talaria
  TranslateTrigger : TuneVar/TranslateTrigger  TriggerInit=[656 270 694 325]
      settings: SourceProductName=Bose Talaria
  Tune Variable : TuneVar/TuneVar  TuneName=FIRCoeffs  SpecifyMaxSize=on  VariableDim=1 (Row)  MaxSize=[maxTotalFirLength 1]  TunabilityNumber=1  MinValue=[]  MaxValue=[]  TriggerInit=[320 375 505 425]  MaskValue=firCoeffsDefault
      settings: SourceProductName=Bose Talaria
  Tune Variable2 : TuneVar/TuneVar  TuneName=PaddedFIRLengths  SpecifyMaxSize=off  VariableDim=1 (Row)  MaxSize=[1 1]  TunabilityNumber=1  MinValue=[]  MaxValue=[]  TriggerInit=[320 470 505 520]  MaskValue=firLengthsDefault
      settings: SourceProductName=Bose Talaria
  translation : MATLAB Function  TreatAsAtomicUnit=on
  wires:
  Tune Variable2/1 -> translation/2(PaddedFIRLengthsIn)  "PaddedFIRLengths"
  translation/2(PaddedFIRLengths) -> TOP2/1
  Tune Variable/1 -> translation/1(FIRCoeffsIn)  "FIRCoeffs"
  TranslateTrigger/1 -> translation/Trigger
  translation/1(FIRCoeffs) -> TOP/1

== system Model_TranslationEngine64/ModelPreAmp/DecRate/Medusa5H1/VLS/VLS Generation - P ==
  FeaturePath : FeaturePath/FeaturePath  FeatureName=GenerationPax  IsGroup=off  GroupNumber=-1  IsModule=off  TriggerInit=[120 244 235 351]
      settings: SourceProductName=Bose Talaria
  TOP : TOP/TOP  TriggerInit=[815 370 985 430]  TopName=FIRCoeffs  DataTypeOut=single  BankNumber=1  PreOverlay=false  PostOverlay=false  Role=Automatic
      settings: SourceProductName=Bose Talaria
  TOP2 : TOP/TOP  TriggerInit=[815 465 985 525]  TopName=PaddedFilterLengths  DataTypeOut=uint32  BankNumber=0  PreOverlay=false  PostOverlay=false  Role=Automatic
      settings: SourceProductName=Bose Talaria
  TranslateTrigger : TuneVar/TranslateTrigger  TriggerInit=[656 270 694 325]
      settings: SourceProductName=Bose Talaria
  Tune Variable : TuneVar/TuneVar  TuneName=FIRCoeffs  SpecifyMaxSize=on  VariableDim=1 (Row)  MaxSize=[maxTotalFirLength 1]  TunabilityNumber=1  MinValue=[]  MaxValue=[]  TriggerInit=[320 375 505 425]  MaskValue=firCoeffsDefault
      settings: SourceProductName=Bose Talaria
  Tune Variable2 : TuneVar/TuneVar  TuneName=PaddedFIRLengths  SpecifyMaxSize=off  VariableDim=1 (Row)  MaxSize=[1 1]  TunabilityNumber=1  MinValue=[]  MaxValue=[]  TriggerInit=[320 470 505 520]  MaskValue=firLengthsDefault
      settings: SourceProductName=Bose Talaria
  translation : MATLAB Function  TreatAsAtomicUnit=on
  wires:
  Tune Variable2/1 -> translation/2(PaddedFIRLengthsIn)  "PaddedFIRLengths"
  translation/2(PaddedFIRLengths) -> TOP2/1
  Tune Variable/1 -> translation/1(FIRCoeffsIn)  "FIRCoeffs"
  TranslateTrigger/1 -> translation/Trigger
  translation/1(FIRCoeffs) -> TOP/1

== system Model_TranslationEngine64/ModelPreAmp/PreAmpPart1/NEARPreAmp/FixedAttenuator/Attenuation  ==
  Function-Call Subsystem : Subsystem  TreatAsAtomicUnit=on
  TOP : TOP/TOP  TriggerInit=[380 164 560 226]  TopName=A  DataTypeOut=single  BankNumber=0  PreOverlay=false  PostOverlay=false  Role=Automatic
      settings: SourceProductName=Bose Talaria
  TranslateTrigger : TuneVar/TranslateTrigger  TriggerInit=[-809 110 -771 165]
      settings: SourceProductName=Bose Talaria
  Tune Variable : TuneVar/TuneVar  TuneName=A  SpecifyMaxSize=off  VariableDim=1 (Row)  MaxSize=[1 1]  TunabilityNumber=1  MinValue=[]  MaxValue=[]  TriggerInit=[-105 164 120 226]  MaskValue=Config.A
      settings: SourceProductName=Bose Talaria
  wires:
  TranslateTrigger/1 -> Function-Call Subsystem/Trigger
  Tune Variable/1 -> Function-Call Subsystem/1(In1)  "A"
  Function-Call Subsystem/1(Out1) -> TOP/1

== system Model_TranslationEngine64/ModelPreAmp/PreAmpPart1/NEARPreAmp/Monoizer/Monoizer ==
  MonoizerStereo : Subsystem  VariantControl=Config.NumChannels == 2
  MonoizerSurround : Subsystem  VariantControl=Config.NumChannels > 2

== system Model_TranslationEngine64/ModelPreAmp/PreAmpPart1/NEARPreAmp/MusicLimiter/annPredTuneTOP ==
  TOP : TOP/TOP  TriggerInit=[440 20 585 80]  TopName=AnnPred  DataTypeOut=single  BankNumber=0  PreOverlay=false  PostOverlay=false  Role=Automatic
      settings: SourceProductName=Bose Talaria
  TranslateTrigger : TuneVar/TranslateTrigger  TriggerInit=[306 -100 344 -45]
      settings: SourceProductName=Bose Talaria
  Trivial Translation : MATLAB Function  TreatAsAtomicUnit=on
  Tune Variable : TuneVar/TuneVar  TuneName=AnnPred  SpecifyMaxSize=off  VariableDim=1 (Row)  MaxSize=[1 1]  TunabilityNumber=1  MinValue=[]  MaxValue=[]  TriggerInit=[20 25 190 75]  MaskValue=Config.TuneDefaults.AnnPred
      settings: SourceProductName=Bose Talaria
  wires:
  TranslateTrigger/1 -> Trivial Translation/Trigger
  Trivial Translation/1(TOP1) -> TOP/1
  Tune Variable/1 -> Trivial Translation/1(Tune1)  "AnnPred"
